simulink model "lab3_model"  (R2015a)
settings: Solver=ode4  StartTime=0.0  StopTime=10.0  FixedStep=1e-2  RelTol=1e-3
values from neighbouring files (symbols this model uses):
  A = 1    [script1.m]
undefined symbols (not defined in the file or in its folder): B, C, D, WPC
settings Model: Creator=bb  LastModifiedBy=bb
settings DataIOCC: LimitDataPoints=off

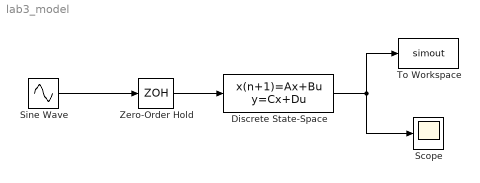
== system lab3_model ==
  Discrete State-Space : DiscreteStateSpace  A=A  B=B  C=C  D=D  X0=WPC
  Scope : Scope
  Sine Wave : Sin  SampleTime=0
  To Workspace : ToWorkspace  VariableName=simout  SaveFormat=Timeseries  SampleTime=-1
  Zero-Order Hold : ZeroOrderHold
  wires:
  Zero-Order Hold/1 -> Discrete State-Space/1
  Discrete State-Space/1 -> To Workspace/1, Scope/1
  Sine Wave/1 -> Zero-Order Hold/1
